simulink model "Exemplu_figura12"  (R2016a)
settings: Solver=VariableStepDiscrete  StartTime=0.0  StopTime=10.0  RelTol=1e-3
undefined symbols (not defined in the file): m, n
settings Model: Creator=Cristina  LastModifiedBy=Cristina

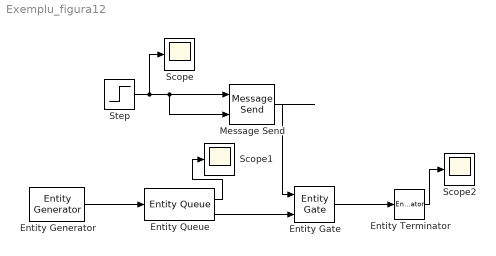
== system Exemplu_figura12 ==
  Entity Gate : EntityGate  InputPortMessageModes=m,m  OutputPortMessageModes=m
  Entity Generator : EntityGenerator  OutputPortMessageModes=m  EntityType=Structured  EntityTypeName=Entity
  Entity Queue : EntityQueue  InputPortMessageModes=m  OutputPortMessageModes=n,m  NumberEntitiesInBlock=on
      settings: OutputPortMap=o1,o5
  Entity Terminator : EntityTerminator  InputPortMessageModes=m  NumberEntitiesArrived=on
      settings: OutputPortMap=o0
  Message Send : MessageSend  OutputPortMessageModes=m  ShowEnablePort=on
      settings: InputPortMap=e0,u1
  Scope : Scope
  Scope1 : Scope
  Scope2 : Scope
  Step : Step  Time=4  SampleTime=0
  wires:
  Step/1 -> Scope/1, Message Send/2, Message Send/1
  Entity Generator/1 -> Entity Queue/1
  Entity Queue/2 -> Entity Gate/2
  Message Send/1 -> Entity Gate/1
  Entity Gate/1 -> Entity Terminator/1
  Entity Queue/1 -> Scope1/1
  Entity Terminator/1 -> Scope2/1
